simulink model "mcpi_loopback_polling_am261"  (R2024b)
settings: Solver=FixedStepAuto  StartTime=0.0  StopTime=10.0  RelTol=1e-3
libraries: peripheral_library_blocks_am261x x6
settings Model: Creator=a0499511  LastModifiedBy=a0499511
settings OptimizationCC: DefaultParameterBehavior=Inlined  EnhancedBackFolding=on  PassReuseOutputArgsAs=Individual arguments  ZeroExternalMemoryAtStartup=off  ZeroInternalMemoryAtStartup=off  MaxStackSize=64  OptimizeBlockOrder=speed  DifferentSizesBufferReuse=on  OptimizationCustomize=off  EfficientTunableParamExpr=on
settings DebuggingCC: ParameterTunabilityLossMsg=error
settings HardwareCC: ProdBitPerPointer=32  ProdBitPerSizeT=32  ProdBitPerPtrDiffT=32  ProdLargestAtomicInteger=Long  ProdLargestAtomicFloat=Double  ProdWordSize=32  ProdHWDeviceType=ARM Compatible->ARM Cortex
settings SFSimCC: MATLABDynamicMemAlloc=off
settings RTWCC: Description=Embedded Coder  SystemTargetFile=ert.tlc  HardwareBoard=AM261X LP  TemplateMakefile=ert_default_tmf  Toolchain=TI ARM Clang Compiler AM261x | gmake
settings CodeAppCC: ForceParamTrailComments=on  IgnoreCustomStorageClasses=off  OperatorAnnotations=on  SimulinkDataObjDesc=on  SFDataObjDesc=on  InsertBlockDesc=on
settings ERTTargetCC: SupportVariableSizeSignals=on  ExtModeTransport=3  ExtModeStaticAlloc=on  ExtModeMexFile=ext_xcp  ExtModeIntrfLevel=Level2 - Open  ERTCustomFileTemplate=AM263x_codertarget_file_process.tlc

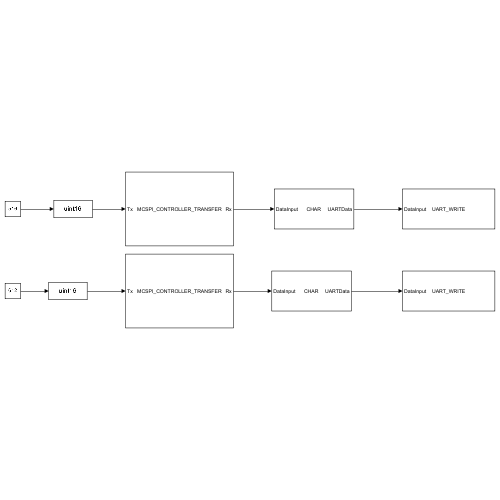
[thumbnail: Simulink's stored preview of the top-level diagram]
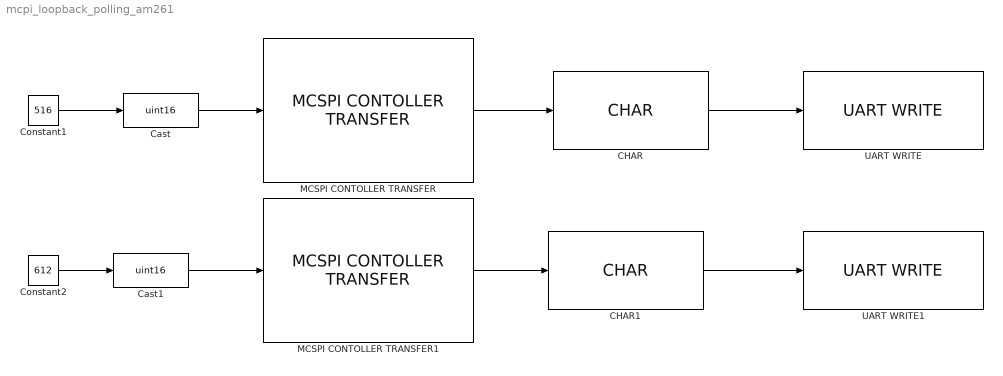
== system mcpi_loopback_polling_am261 ==
  CHAR : peripheral_library_blocks_am261x/CHAR
  CHAR1 : peripheral_library_blocks_am261x/CHAR
  Cast : DataTypeConversion  OutDataTypeStr=uint16  SaturateOnIntegerOverflow=off  RndMeth=Floor
  Cast1 : DataTypeConversion  OutDataTypeStr=uint16  SaturateOnIntegerOverflow=off  RndMeth=Floor
  Constant1 : Constant  Value=516
  Constant2 : Constant  Value=612
  MCSPI CONTOLLER TRANSFER : peripheral_library_blocks_am261x/MCSPI CONTOLLER TRANSFER  MCSPI_Instance=MCSPI0  Enable_Channel0=on  Enable_Channel1=off  Output_Data_Length=1  Channel0_Data_Size=8  Channel0_Auto_CSDeassert=on  Channel1_Data_Size=8  Channel1_Auto_CSDeassert=on
  MCSPI CONTOLLER TRANSFER1 : peripheral_library_blocks_am261x/MCSPI CONTOLLER TRANSFER  MCSPI_Instance=MCSPI0  Enable_Channel0=on  Enable_Channel1=off  Output_Data_Length=1  Channel0_Data_Size=8  Channel0_Auto_CSDeassert=on  Channel1_Data_Size=8  Channel1_Auto_CSDeassert=on
  UART WRITE : peripheral_library_blocks_am261x/UART WRITE  UARTPort=UART0
  UART WRITE1 : peripheral_library_blocks_am261x/UART WRITE  UARTPort=UART0
  wires:
  Constant2/1 -> Cast1/1
  Cast1/1 -> MCSPI CONTOLLER TRANSFER1/1
  CHAR1/1 -> UART WRITE1/1
  Cast/1 -> MCSPI CONTOLLER TRANSFER/1
  MCSPI CONTOLLER TRANSFER1/1 -> CHAR1/1
  Constant1/1 -> Cast/1
  MCSPI CONTOLLER TRANSFER/1 -> CHAR/1
  CHAR/1 -> UART WRITE/1
